simulink model "FW_LinLongitudinalModel"  (R2020a)
settings: Solver=ode45  StartTime=0.0  StopTime=Trun  RelTol=1e-3  EnableMultiTasking=on
model workspace (MAT data in the model file):
  Initial_Long_roll = 0
undefined symbols (not defined in the file): Initial_Lat, Mdel_e, Mq, Mu, Mw, Tr_psi, Tr_q, Tr_theta, Tr_u, Tr_w, Xdel_e, Xdel_t, Xq, Xu, Xw, Zdel_e, Zq, Zu, Zw
settings Model: Creator=user  LastModifiedBy=patel
settings DataIOCC: LimitDataPoints=on  SaveFormat=Array  ReturnWorkspaceOutputs=off
settings OptimizationCC: LifeSpan=inf
settings DebuggingCC: SFUnexpectedBacktrackingDiag=warning  SFNoUnconditionalDefaultTransitionDiag=warning  SFExecutionAtInitializationDiag=none  ArithmeticOperatorsInVariantConditions=warning
settings HardwareCC: ProdBitPerPointer=32  ProdBitPerSizeT=32  ProdBitPerPtrDiffT=32  ProdLargestAtomicFloat=None  ProdIntDivRoundTo=Undefined  ProdEndianess=Unspecified  ProdWordSize=32  ProdHWDeviceType=32-bit Generic
settings ModelReferenceCC: PropagateSignalLabelsOutOfModel=off
settings SFSimCC: SimUseLocalCustomCode=off  CustomCodeUndefinedFunction=UseInterfaceOnly
settings RTWCC: RTWUseLocalCustomCode=off
settings CodeAppCC: StateflowObjectComments=on
settings GRTTargetCC: TargetLangStandard=C89/C90 (ANSI)
settings ConfigComp: CovMetricSettings=dw  CovHtmlReporting=on  CovSaveCumulativeToWorkspaceVar=on  CovSaveSingleToWorkspaceVar=on  CovExternalEMLEnable=off

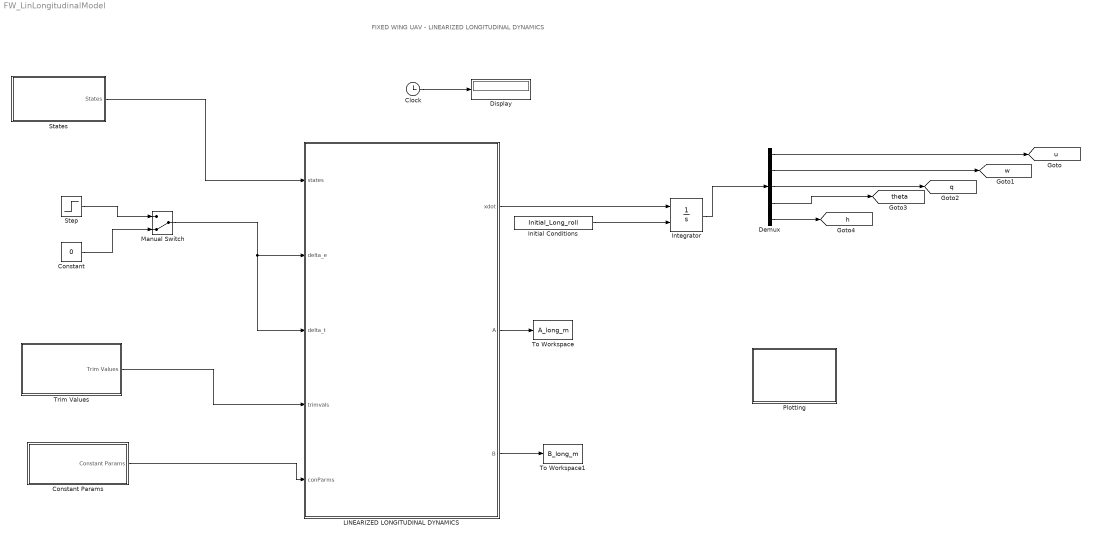
== system FW_LinLongitudinalModel ==
  note: FIXED WING UAV - LINEARIZED LONGITUDINAL DYNAMICS
  Clock : Clock
  Constant : Constant  Value=0
  Constant Params : Subsystem
  Demux : Demux  Outputs=5
  Display : Display
  Initial Conditions : Constant  Value=Initial_Long_roll
  Integrator : Integrator  InitialConditionSource=external  InitialCondition=Initial_Lat
  LINEARIZED LONGITUDINAL DYNAMICS : MATLAB Function  TreatAsAtomicUnit=on
  Manual Switch : ManualSwitch  CurrentSetting=0
  Plotting : Subsystem
  States : Subsystem
  Step : Step  SampleTime=0
  To Workspace : ToWorkspace  VariableName=A_long_m  SampleTime=-1
      settings: MaxDataPoints=1
  To Workspace1 : ToWorkspace  VariableName=B_long_m  SampleTime=-1
      settings: MaxDataPoints=1
  Trim Values : Subsystem
  tag scope: h=global, q=global, theta=global, u=global, w=global
  wires:
  LINEARIZED LONGITUDINAL DYNAMICS/1(xdot) -> Integrator/1
  LINEARIZED LONGITUDINAL DYNAMICS/3(B) -> To Workspace1/1
  Integrator/1 -> Demux/1
  Demux/1 -> [u]
  Demux/2 -> [w]
  Demux/3 -> [q]
  Demux/4 -> [theta]
  Demux/5 -> [h]
  States/1(States) -> LINEARIZED LONGITUDINAL DYNAMICS/1(states)
  LINEARIZED LONGITUDINAL DYNAMICS/2(A) -> To Workspace/1
  Trim Values/1(Trim Values) -> LINEARIZED LONGITUDINAL DYNAMICS/4(trimvals)
  Constant Params/1("Constant Params ") -> LINEARIZED LONGITUDINAL DYNAMICS/5(conParms)
  Clock/1 -> Display/1
  Step/1 -> Manual Switch/1
  Constant/1 -> Manual Switch/2
  Manual Switch/1 -> LINEARIZED LONGITUDINAL DYNAMICS/3(delta_t), LINEARIZED LONGITUDINAL DYNAMICS/2(delta_e)
  Initial Conditions/1 -> Integrator/2

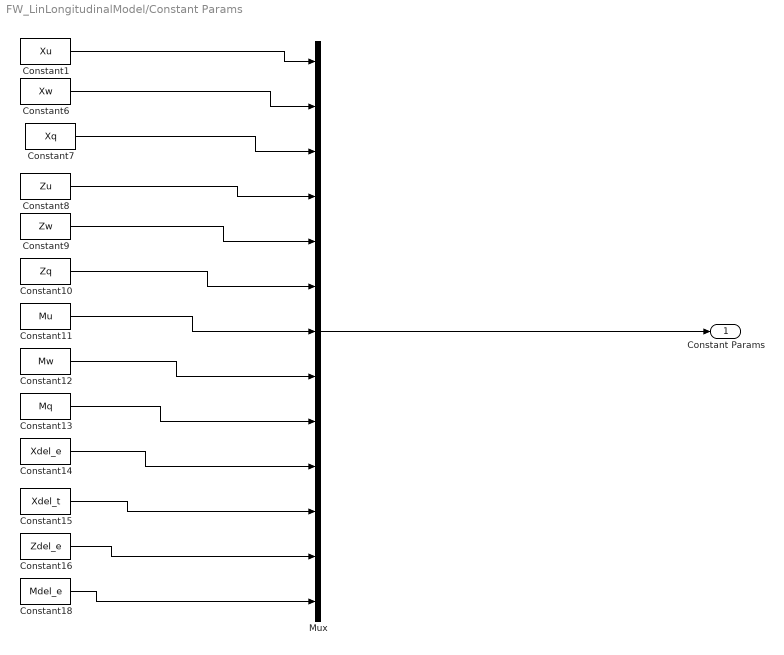
== system FW_LinLongitudinalModel/Constant Params ==
  Constant1 : Constant  Value=Xu
  Constant10 : Constant  Value=Zq
  Constant11 : Constant  Value=Mu
  Constant12 : Constant  Value=Mw
  Constant13 : Constant  Value=Mq
  Constant14 : Constant  Value=Xdel_e
  Constant15 : Constant  Value=Xdel_t
  Constant16 : Constant  Value=Zdel_e
  Constant18 : Constant  Value=Mdel_e
  Constant6 : Constant  Value=Xw
  Constant7 : Constant  Value=Xq
  Constant8 : Constant  Value=Zu
  Constant9 : Constant  Value=Zw
  Mux : Mux  Inputs=13
  "Constant Params " : Outport
  wires:
  Constant14/1 -> Mux/10
  Constant15/1 -> Mux/11
  Constant18/1 -> Mux/13
  Constant16/1 -> Mux/12
  Constant6/1 -> Mux/2
  Constant7/1 -> Mux/3
  Constant13/1 -> Mux/9
  Constant10/1 -> Mux/6
  Constant8/1 -> Mux/4
  Constant9/1 -> Mux/5
  Constant11/1 -> Mux/7
  Constant12/1 -> Mux/8
  Mux/1 -> "Constant Params "/1
  Constant1/1 -> Mux/1

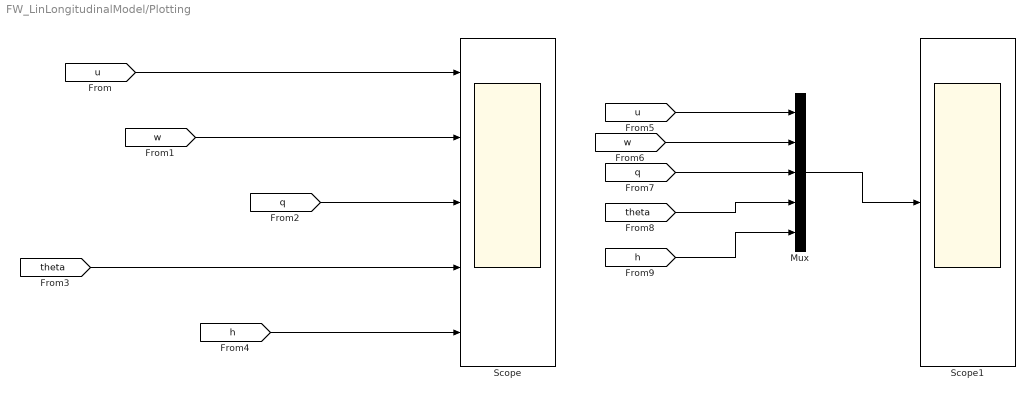
== system FW_LinLongitudinalModel/Plotting ==
  Mux : Mux  Inputs=5
  Scope : Scope  NumInputPorts=5
  Scope1 : Scope
  wires:
  [theta] -> Scope/4
  [w] -> Scope/2
  [h] -> Scope/5
  [u] -> Scope/1
  [q] -> Scope/3
  [u] -> Mux/1
  [w] -> Mux/2
  [q] -> Mux/3
  [theta] -> Mux/4
  [h] -> Mux/5
  Mux/1 -> Scope1/1

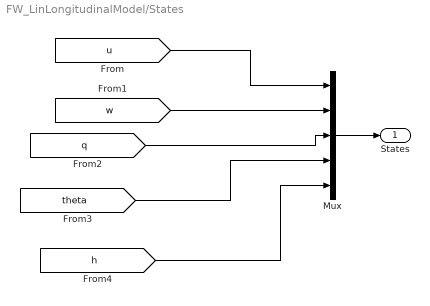
== system FW_LinLongitudinalModel/States ==
  Mux : Mux  Inputs=5
  States : Outport  PortDimensions=5
  wires:
  [q] -> Mux/3
  [theta] -> Mux/4
  [h] -> Mux/5
  Mux/1 -> States/1
  [u] -> Mux/1
  [w] -> Mux/2

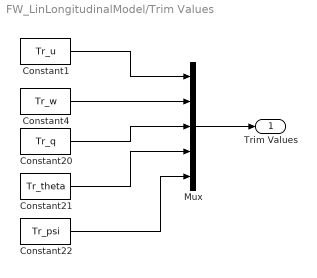
== system FW_LinLongitudinalModel/Trim Values ==
  Constant1 : Constant  Value=Tr_u
  Constant20 : Constant  Value=Tr_q
  Constant21 : Constant  Value=Tr_theta
  Constant22 : Constant  Value=Tr_psi
  Constant4 : Constant  Value=Tr_w
  Mux : Mux  Inputs=5
  Trim Values : Outport  PortDimensions=5
  wires:
  Constant4/1 -> Mux/2
  Mux/1 -> Trim Values/1
  Constant1/1 -> Mux/1
  Constant21/1 -> Mux/4
  Constant20/1 -> Mux/3
  Constant22/1 -> Mux/5

== matlab function FW_LinLongitudinalModel/LINEARIZED LONGITUDINAL DYNAMICS ==
  data: states input; xdot output; delta_e input; delta_t input; A output; B output; trimvals input; conParms input
function [xdot,A,B] = Linearized_Logitudinal_Dynamics(states,delta_e,delta_t,trimvals,conParms)
%% LINEARIZED LONGITUDINAL DYNAMICS
% States: [u,w,q,theta,h]
% Inputs:  [del_e,del_t]
% Paramters used
% P : Paramters of the system
% Tr : Trim Values
gravity = 9.81;
%% States
u = states(1);
w =states(2);
q = states(3);
theta =states(4);
h = states(5);
%% Trim Values
Tr_u=trimvals(1);
Tr_w=trimvals(2);
Tr_q=trimvals(3);
Tr_theta=trimvals(4);
Tr_h=trimvals(5);
%% Constant Parameter
Xu=conParms(1);
Xw=conParms(2);
Xq=conParms(3);
Zu=conParms(4);
Zw=conParms(5);
Zq=conParms(6);
Mu=conParms(7);
Mw=conParms(8);
Mq=conParms(9);
Xdel_e=conParms(10);
Xdel_t=conParms(11);
Zdel_e=conParms(12);
Mdel_e=conParms(13);
%---------------------------------------
%  State Space Matrices
A = [Xu Xw Xq -gravity*cos(Tr_theta) 0;
     Zu Zw Zq -gravity*sin(Tr_theta) 0;
     Mu Mw Mq 0 0;
     0 0 1  0 0;
     sin(Tr_theta) -cos(Tr_theta) 0 Tr_u*cos(Tr_theta)+Tr_w*sin(Tr_theta) 0];
 
B  = [Xdel_e Xdel_t; 
      Zdel_e 0;
      Mdel_e 0;
      0 0;
      0 0];

x = [u;w;q;theta;h];
u = [delta_e;delta_t];

xdot = A*x + B*u;


% Longitudinal State Space Model
